simulink model "temp_c2f"  (R2019a)
settings: Solver=VariableStepAuto  StartTime=0.0  StopTime=10.0  RelTol=1e-3
settings Model: Creator=rosha  LastModifiedBy=rosha

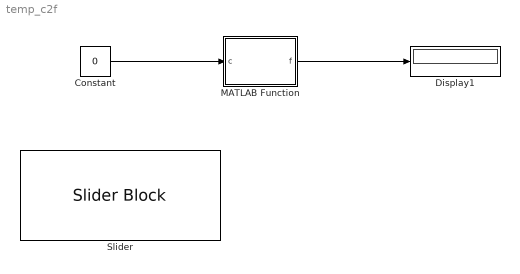
== system temp_c2f ==
  Constant : Constant  Value=0
  Display1 : Display
  MATLAB Function : MATLAB Function  TreatAsAtomicUnit=on
  Slider : SliderBlock
  wires:
  MATLAB Function/1(f) -> Display1/1
  Constant/1 -> MATLAB Function/1(c)

== matlab function temp_c2f/MATLAB Function ==
  data: c input; f output
function f = fcn(c)

f = (c * (9/5)) + 32;
